simulink model "automata_learning"  (R2022a)
(part 10 of 10)

0.6710054278373718) + 1.0) + 0.26810726523399353 * (exp(0.6629329919815063 * x1 - 0.3119186460971832 * x2 + 0.20862619578838348) - 1.0) / (exp(0.6629329919815063 * x1 - 0.3119186460971832 * x2 + 0.20862619578838348) + 1.0) + 0.9232311844825745 * (exp(0.6406594514846802 * x1 + 0.05703261122107506 * x2 + 0.3176595866680145) - 1.0) / (exp(0.6406594514846802 * x1 + 0.05703261122107506 * x2 + 0.3176595866680145) + 1.0) + 0.7681644558906555 * (exp(0.9188533425331116 * x1 + 0.3101022243499756 * x2 + 0.6654399037361145) - 1.0) / (exp(0.9188533425331116 * x1 + 0.3101022243499756 * x2 + 0.6654399037361145) + 1.0) - 0.2590520679950714 * (exp(0.575993537902832 * x1 - 0.4726734459400177 * x2 + 0.7029635310173035) - 1.0) / (exp(0.575993537902832 * x1 - 0.4726734459400177 * x2 + 0.7029635310173035) + 1.0) + 0.9095823168754578 * (exp(0.7590878009796143 * x1 - 0.23670220375061035 * x2 + 1.0534344911575317) - 1.0) / (exp(0.7590878009796143 * x1 - 0.23670220375061035 * x2 + 1.0534344911575317) + 1.0) + 0.7333047389984131 * (exp(0.5151293277740479 * x1 - 0.39795804023742676 * x2 + 0.11806197464466095) - 1.0) / (exp(0.5151293277740479 * x1 - 0.39795804023742676 * x2 + 0.11806197464466095) + 1.0) + 0.9102956652641296 * (exp(0.4433993697166443 * x1 - 0.08205956220626831 * x2 + 0.18252399563789368) - 1.0) / (exp(0.4433993697166443 * x1 - 0.08205956220626831 * x2 + 0.18252399563789368) + 1.0) + 0.8548353910446167 * (exp(0.48641395568847656 * x1 + 0.8826764822006226 * x2 + 0.5417870879173279) - 1.0) / (exp(0.48641395568847656 * x1 + 0.8826764822006226 * x2 + 0.5417870879173279) + 1.0) + 0.536832332611084 * (exp(0.47229835391044617 * x1 - 0.20287995040416718 * x2 + 0.34894588589668274) - 1.0) / (exp(0.47229835391044617 * x1 - 0.20287995040416718 * x2 + 0.34894588589668274) + 1.0) + 0.24342596530914307) + 1.0) + 0.9671072959899902 * (exp(0.5794932246208191 * (exp(0.55704265832901 * x1 + 0.592957079410553 * x2 + 0.33553701639175415) - 1.0) / (exp(0.55704265832901 * x1 + 0.592957079410553 * x2 + 0.33553701639175415) + 1.0) + 0.9518229365348816 * (exp(0.6549424529075623 * x1 - 0.1391940712928772 * x2 + 0.6311511397361755) - 1.0) / (exp(0.6549424529075623 * x1 - 0.1391940712928772 * x2 + 0.6311511397361755) + 1.0) + 0.44287005066871643 * (exp(0.6888914704322815 * x1 - 0.6110755205154419 * x2 + 0.6041516661643982) - 1.0) / (exp(0.6888914704322815 * x1 - 0.6110755205154419 * x2 + 0.6041516661643982) + 1.0) + 0.6187660694122314 * (exp(0.20129768550395966 * x2 - 1.0647046566009521 * x1 + 0.5778789520263672) - 1.0) / (exp(0.20129768550395966 * x2 - 1.0647046566009521 * x1 + 0.5778789520263672) + 1.0) - 0.48944976925849915 * (exp(0.07980049401521683 * x1 + 0.6124646663665771 * x2 - 0.1684141308069229) - 1.0) / (exp(0.07980049401521683 * x1 + 0.6124646663665771 * x2 - 0.1684141308069229) + 1.0) + 0.1713249534368515 * (exp(0.361889123916626 * x1 + 0.6644142866134644 * x2 + 0.2823045253753662) - 1.0) / (exp(0.361889123916626 * x1 + 0.6644142866134644 * x2 + 0.2823045253753662) + 1.0) - 0.9707628488540649 * (exp(0.6355613470077515 * x1 + 0.7923728823661804 * x2 + 0.27106547355651855) - 1.0) / (exp(0.6355613470077515 * x1 + 0.7923728823661804 * x2 + 0.27106547355651855) + 1.0) + 0.23367302119731903 * (exp(0.2957508862018585 * x1 + 0.41109827160835266 * x2 + 0.13971224427223206) - 1.0) / (exp(0.2957508862018585 * x1 + 0.41109827160835266 * x2 + 0.13971224427223206) + 1.0) - 1.041667103767395 * (exp(0.7331780195236206 * x1 + 1.0149563550949097 * x2 - 0.37788793444633484) - 1.0) / (exp(0.7331780195236206 * x1 + 1.0149563550949097 * x2 - 0.37788793444633484) + 1.0) + 0.5859559774398804 * (exp(0.6101927757263184 * x1 - 0.32282912731170654 * x2 + 0.7518836855888367) - 1.0) / (exp(0.6101927757263184 * x1 - 0.32282912731170654 * x2 + 0.7518836855888367) + 1.0) + 0.6447692513465881 * (exp(0.2542825937271118 * x1 + 0.9084843397140503 * x2 + 0.6710054278373718) - 1.0) / (exp(0.2542825937271118 * x1 + 0.9084843397140503 * x2 + 0.6710054278373718) + 1.0) + 0.8346514701843262 * (exp(0.6629329919815063 * x1 - 0.3119186460971832 * x2 + 0.20862619578838348) - 1.0) / (exp(0.6629329919815063 * x1 - 0.3119186460971832 * x2 + 0.20862619578838348) + 1.0) - 0.11273422837257385 * (exp(0.6406594514846802 * x1 + 0.05703261122107506 * x2 + 0.3176595866680145) - 1.0) / (exp(0.6406594514846802 * x1 + 0.05703261122107506 * x2 + 0.3176595866680145) + 1.0) + 1.3257321119308472 * (exp(0.9188533425331116 * x1 + 0.3101022243499756 * x2 + 0.6654399037361145) - 1.0) / (exp(0.9188533425331116 * x1 + 0.3101022243499756 * x2 + 0.6654399037361145) + 1.0) + 0.364542692899704 * (exp(0.575993537902832 * x1 - 0.4726734459400177 * x2 + 0.7029635310173035) - 1.0) / (exp(0.575993537902832 * x1 - 0.4726734459400177 * x2 + 0.7029635310173035) + 1.0) + 1.3769431114196777 * (exp(0.7590878009796143 * x1 - 0.23670220375061035 * x2 + 1.0534344911575317) - 1.0) / (exp(0.7590878009796143 * x1 - 0.23670220375061035 * x2 + 1.0534344911575317) + 1.0) + 0.25804296135902405 * (exp(0.5151293277740479 * x1 - 0.39795804023742676 * x2 + 0.11806197464466095) - 1.0) / (exp(0.5151293277740479 * x1 - 0.39795804023742676 * x2 + 0.11806197464466095) + 1.0) + 0.17459556460380554 * (exp(0.4433993697166443 * x1 - 0.08205956220626831 * x2 + 0.18252399563789368) - 1.0) / (exp(0.4433993697166443 * x1 - 0.08205956220626831 * x2 + 0.18252399563789368) + 1.0) + 0.7206000089645386 * (exp(0.48641395568847656 * x1 + 0.8826764822006226 * x2 + 0.5417870879173279) - 1.0) / (exp(0.48641395568847656 * x1 + 0.8826764822006226 * x2 + 0.5417870879173279) + 1.0) + 0.03906390815973282 * (exp(0.47229835391044617 * x1 - 0.20287995040416718 * x2 + 0.34894588589668274) - 1.0) / (exp(0.47229835391044617 * x1 - 0.20287995040416718 * x2 + 0.34894588589668274) + 1.0) + 0.22301727533340454) - 1.0) / (exp(0.5794932246208191 * (exp(0.55704265832901 * x1 + 0.592957079410553 * x2 + 0.33553701639175415) - 1.0) / (exp(0.55704265832901 * x1 + 0.592957079410553 * x2 + 0.33553701639175415) + 1.0) + 0.9518229365348816 * (exp(0.6549424529075623 * x1 - 0.1391940712928772 * x2 + 0.6311511397361755) - 1.0) / (exp(0.6549424529075623 * x1 - 0.1391940712928772 * x2 + 0.6311511397361755) + 1.0) + 0.44287005066871643 * (exp(0.6888914704322815 * x1 - 0.6110755205154419 * x2 + 0.6041516661643982) - 1.0) / (exp(0.6888914704322815 * x1 - 0.6110755205154419 * x2 + 0.6041516661643982) + 1.0) + 0.6187660694122314 * (exp(0.20129768550395966 * x2 - 1.0647046566009521 * x1 + 0.5778789520263672) - 1.0) / (exp(0.20129768550395966 * x2 - 1.0647046566009521 * x1 + 0.5778789520263672) + 1.0) - 0.48944976925849915 * (exp(0.07980049401521683 * x1 + 0.6124646663665771 * x2 - 0.1684141308069229) - 1.0) / (exp(0.07980049401521683 * x1 + 0.6124646663665771 * x2 - 0.1684141308069229) + 1.0) + 0.1713249534368515 * (exp(0.361889123916626 * x1 + 0.6644142866134644 * x2 + 0.2823045253753662) - 1.0) / (exp(0.361889123916626 * x1 + 0.6644142866134644 * x2 + 0.2823045253753662) + 1.0) - 0.9707628488540649 * (exp(0.6355613470077515 * x1 + 0.7923728823661804 * x2 + 0.27106547355651855) - 1.0) / (exp(0.6355613470077515 * x1 + 0.7923728823661804 * x2 + 0.27106547355651855) + 1.0) + 0.23367302119731903 * (exp(0.2957508862018585 * x1 + 0.41109827160835266 * x2 + 0.13971224427223206) - 1.0) / (exp(0.2957508862018585 * x1 + 0.41109827160835266 * x2 + 0.13971224427223206) + 1.0) - 1.041667103767395 * (exp(0.7331780195236206 * x1 + 1.0149563550949097 * x2 - 0.37788793444633484) - 1.0) / (exp(0.7331780195236206 * x1 + 1.0149563550949097 * x2 - 0.37788793444633484) + 1.0) + 0.5859559774398804 * (exp(0.6101927757263184 * x1 - 0.32282912731170654 * x2 + 0.7518836855888367) - 1.0) / (exp(0.6101927757263184 * x1 - 0.32282912731170654 * x2 + 0.7518836855888367) + 1.0) + 0.6447692513465881 * (exp(0.2542825937271118 * x1 + 0.9084843397140503 * x2 + 0.6710054278373718) - 1.0) / (exp(0.2542825937271118 * x1 + 0.9084843397140503 * x2 + 0.6710054278373718) + 1.0) + 0.8346514701843262 * (exp(0.6629329919815063 * x1 - 0.3119186460971832 * x2 + 0.20862619578838348) - 1.0) / (exp(0.6629329919815063 * x1 - 0.3119186460971832 * x2 + 0.20862619578838348) + 1.0) - 0.11273422837257385 * (exp(0.6406594514846802 * x1 + 0.05703261122107506 * x2 + 0.3176595866680145) - 1.0) / (exp(0.6406594514846802 * x1 + 0.05703261122107506 * x2 + 0.3176595866680145) + 1.0) + 1.3257321119308472 * (exp(0.9188533425331116 * x1 + 0.3101022243499756 * x2 + 0.6654399037361145) - 1.0) / (exp(0.9188533425331116 * x1 + 0.3101022243499756 * x2 + 0.6654399037361145) + 1.0) + 0.364542692899704 * (exp(0.575993537902832 * x1 - 0.4726734459400177 * x2 + 0.7029635310173035) - 1.0) / (exp(0.575993537902832 * x1 - 0.4726734459400177 * x2 + 0.7029635310173035) + 1.0) + 1.3769431114196777 * (exp(0.7590878009796143 * x1 - 0.23670220375061035 * x2 + 1.0534344911575317) - 1.0) / (exp(0.7590878009796143 * x1 - 0.23670220375061035 * x2 + 1.0534344911575317) + 1.0) + 0.25804296135902405 * (exp(0.5151293277740479 * x1 - 0.39795804023742676 * x2 + 0.11806197464466095) - 1.0) / (exp(0.5151293277740479 * x1 - 0.39795804023742676 * x2 + 0.11806197464466095) + 1.0) + 0.17459556460380554 * (exp(0.4433993697166443 * x1 - 0.08205956220626831 * x2 + 0.18252399563789368) - 1.0) / (exp(0.4433993697166443 * x1 - 0.08205956220626831 * x2 + 0.18252399563789368) + 1.0) + 0.7206000089645386 * (exp(0.48641395568847656 * x1 + 0.8826764822006226 * x2 + 0.5417870879173279) - 1.0) / (exp(0.48641395568847656 * x1 + 0.8826764822006226 * x2 + 0.5417870879173279) + 1.0) + 0.03906390815973282 * (exp(0.47229835391044617 * x1 - 0.20287995040416718 * x2 + 0.34894588589668274) - 1.0) / (exp(0.47229835391044617 * x1 - 0.20287995040416718 * x2 + 0.34894588589668274) + 1.0) + 0.22301727533340454) + 1.0) + 0.44379422068595886 * (exp(0.004474600311368704 * (exp(0.6549424529075623 * x1 - 0.1391940712928772 * x2 + 0.6311511397361755) - 1.0) / (exp(0.6549424529075623 * x1 - 0.1391940712928772 * x2 + 0.6311511397361755) + 1.0) - 0.22987298667430878 * (exp(0.55704265832901 * x1 + 0.592957079410553 * x2 + 0.33553701639175415) - 1.0) / (exp(0.55704265832901 * x1 + 0.592957079410553 * x2 + 0.33553701639175415) + 1.0) + 0.6058520674705505 * (exp(0.6888914704322815 * x1 - 0.6110755205154419 * x2 + 0.6041516661643982) - 1.0) / (exp(0.6888914704322815 * x1 - 0.6110755205154419 * x2 + 0.6041516661643982) + 1.0) - 1.357459306716919 * (exp(0.20129768550395966 * x2 - 1.0647046566009521 * x1 + 0.5778789520263672) - 1.0) / (exp(0.20129768550395966 * x2 - 1.0647046566009521 * x1 + 0.5778789520263672) + 1.0) - 0.15493887662887573 * (exp(0.07980049401521683 * x1 + 0.6124646663665771 * x2 - 0.1684141308069229) - 1.0) / (exp(0.07980049401521683 * x1 + 0.6124646663665771 * x2 - 0.1684141308069229) + 1.0) + 0.5729637742042542 * (exp(0.361889123916626 * x1 + 0.6644142866134644 * x2 + 0.2823045253753662) - 1.0) / (exp(0.361889123916626 * x1 + 0.6644142866134644 * x2 + 0.2823045253753662) + 1.0) + 0.14763222634792328 * (exp(0.6355613470077515 * x1 + 0.7923728823661804 * x2 + 0.27106547355651855) - 1.0) / (exp(0.6355613470077515 * x1 + 0.7923728823661804 * x2 + 0.27106547355651855) + 1.0) + 0.9889805912971497 * (exp(0.2957508862018585 * x1 + 0.41109827160835266 * x2 + 0.13971224427223206) - 1.0) / (exp(0.2957508862018585 * x1 + 0.41109827160835266 * x2 + 0.13971224427223206) + 1.0) - 0.027431178838014603 * (exp(0.7331780195236206 * x1 + 1.0149563550949097 * x2 - 0.37788793444633484) - 1.0) / (exp(0.7331780195236206 * x1 + 1.0149563550949097 * x2 - 0.37788793444633484) + 1.0) - 0.22922979295253754 * (exp(0.6101927757263184 * x1 - 0.32282912731170654 * x2 + 0.7518836855888367) - 1.0) / (exp(0.6101927757263184 * x1 - 0.32282912731170654 * x2 + 0.7518836855888367) + 1.0) + 0.16280798614025116 * (exp(0.2542825937271118 * x1 + 0.9084843397140503 * x2 + 0.6710054278373718) - 1.0) / (exp(0.2542825937271118 * x1 + 0.9084843397140503 * x2 + 0.6710054278373718) + 1.0) + 0.3429515063762665 * (exp(0.6629329919815063 * x1 - 0.3119186460971832 * x2 + 0.20862619578838348) - 1.0) / (exp(0.6629329919815063 * x1 - 0.3119186460971832 * x2 + 0.20862619578838348) + 1.0) + 1.2585675716400146 * (exp(0.6406594514846802 * x1 + 0.05703261122107506 * x2 + 0.3176595866680145) - 1.0) / (exp(0.6406594514846802 * x1 + 0.05703261122107506 * x2 + 0.3176595866680145) + 1.0) + 0.7193031311035156 * (exp(0.9188533425331116 * x1 + 0.3101022243499756 * x2 + 0.6654399037361145) - 1.0) / (exp(0.9188533425331116 * x1 + 0.3101022243499756 * x2 + 0.6654399037361145) + 1.0) + 0.42601025104522705 * (exp(0.575993537902832 * x1 - 0.4726734459400177 * x2 + 0.7029635310173035) - 1.0) / (exp(0.575993537902832 * x1 - 0.4726734459400177 * x2 + 0.7029635310173035) + 1.0) + 0.8000105023384094 * (exp(0.7590878009796143 * x1 - 0.23670220375061035 * x2 + 1.0534344911575317) - 1.0) / (exp(0.7590878009796143 * x1 - 0.23670220375061035 * x2 + 1.0534344911575317) + 1.0) + 0.8869855999946594 * (exp(0.5151293277740479 * x1 - 0.39795804023742676 * x2 + 0.11806197464466095) - 1.0) / (exp(0.5151293277740479 * x1 - 0.39795804023742676 * x2 + 0.11806197464466095) + 1.0) + 0.6011543273925781 * (exp(0.4433993697166443 * x1 - 0.08205956220626831 * x2 + 0.18252399563789368) - 1.0) / (exp(0.4433993697166443 * x1 - 0.08205956220626831 * x2 + 0.18252399563789368) + 1.0) - 0.04096032679080963 * (exp(0.48641395568847656 * x1 + 0.8826764822006226 * x2 + 0.5417870879173279) - 1.0) / (exp(0.48641395568847656 * x1 + 0.8826764822006226 * x2 + 0.5417870879173279) + 1.0) + 0.8472379446029663 * (exp(0.47229835391044617 * x1 - 0.20287995040416718 * x2 + 0.34894588589668274) - 1.0) / (exp(0.47229835391044617 * x1 - 0.20287995040416718 * x2 + 0.34894588589668274) + 1.0) - 0.481460839509964) - 1.0) / (exp(0.004474600311368704 * (exp(0.6549424529075623 * x1 - 0.1391940712928772 * x2 + 0.6311511397361755) - 1.0) / (exp(0.6549424529075623 * x1 - 0.1391940712928772 * x2 + 0.6311511397361755) + 1.0) - 0.22987298667430878 * (exp(0.55704265832901 * x1 + 0.592957079410553 * x2 + 0.33553701639175415) - 1.0) / (exp(0.55704265832901 * x1 + 0.592957079410553 * x2 + 0.33553701639175415) + 1.0) + 0.6058520674705505 * (exp(0.6888914704322815 * x1 - 0.6110755205154419 * x2 + 0.6041516661643982) - 1.0) / (exp(0.6888914704322815 * x1 - 0.6110755205154419 * x2 + 0.6041516661643982) + 1.0) - 1.357459306716919 * (exp(0.20129768550395966 * x2 - 1.0647046566009521 * x1 + 0.5778789520263672) - 1.0) / (exp(0.20129768550395966 * x2 - 1.0647046566009521 * x1 + 0.5778789520263672) + 1.0) - 0.15493887662887573 * (exp(0.07980049401521683 * x1 + 0.6124646663665771 * x2 - 0.1684141308069229) - 1.0) / (exp(0.07980049401521683 * x1 + 0.6124646663665771 * x2 - 0.1684141308069229) + 1.0) + 0.5729637742042542 * (exp(0.361889123916626 * x1 + 0.6644142866134644 * x2 + 0.2823045253753662) - 1.0) / (exp(0.361889123916626 * x1 + 0.6644142866134644 * x2 + 0.2823045253753662) + 1.0) + 0.14763222634792328 * (exp(0.6355613470077515 * x1 + 0.7923728823661804 * x2 + 0.27106547355651855) - 1.0) / (exp(0.6355613470077515 * x1 + 0.7923728823661804 * x2 + 0.27106547355651855) + 1.0) + 0.9889805912971497 * (exp(0.2957508862018585 * x1 + 0.41109827160835266 * x2 + 0.13971224427223206) - 1.0) / (exp(0.2957508862018585 * x1 + 0.41109827160835266 * x2 + 0.13971224427223206) + 1.0) - 0.027431178838014603 * (exp(0.7331780195236206 * x1 + 1.0149563550949097 * x2 - 0.37788793444633484) - 1.0) / (exp(0.7331780195236206 * x1 + 1.0149563550949097 * x2 - 0.37788793444633484) + 1.0) - 0.22922979295253754 * (exp(0.6101927757263184 * x1 - 0.32282912731170654 * x2 + 0.7518836855888367) - 1.0) / (exp(0.6101927757263184 * x1 - 0.32282912731170654 * x2 + 0.7518836855888367) + 1.0) + 0.16280798614025116 * (exp(0.2542825937271118 * x1 + 0.9084843397140503 * x2 + 0.6710054278373718) - 1.0) / (exp(0.2542825937271118 * x1 + 0.9084843397140503 * x2 + 0.6710054278373718) + 1.0) + 0.3429515063762665 * (exp(0.6629329919815063 * x1 - 0.3119186460971832 * x2 + 0.20862619578838348) - 1.0) / (exp(0.6629329919815063 * x1 - 0.3119186460971832 * x2 + 0.20862619578838348) + 1.0) + 1.2585675716400146 * (exp(0.6406594514846802 * x1 + 0.05703261122107506 * x2 + 0.3176595866680145) - 1.0) / (exp(0.6406594514846802 * x1 + 0.05703261122107506 * x2 + 0.3176595866680145) + 1.0) + 0.7193031311035156 * (exp(0.9188533425331116 * x1 + 0.3101022243499756 * x2 + 0.6654399037361145) - 1.0) / (exp(0.9188533425331116 * x1 + 0.3101022243499756 * x2 + 0.6654399037361145) + 1.0) + 0.42601025104522705 * (exp(0.575993537902832 * x1 - 0.4726734459400177 * x2 + 0.7029635310173035) - 1.0) / (exp(0.575993537902832 * x1 - 0.4726734459400177 * x2 + 0.7029635310173035) + 1.0) + 0.8000105023384094 * (exp(0.7590878009796143 * x1 - 0.23670220375061035 * x2 + 1.0534344911575317) - 1.0) / (exp(0.7590878009796143 * x1 - 0.23670220375061035 * x2 + 1.0534344911575317) + 1.0) + 0.8869855999946594 * (exp(0.5151293277740479 * x1 - 0.39795804023742676 * x2 + 0.11806197464466095) - 1.0) / (exp(0.5151293277740479 * x1 - 0.39795804023742676 * x2 + 0.11806197464466095) + 1.0) + 0.6011543273925781 * (exp(0.4433993697166443 * x1 - 0.08205956220626831 * x2 + 0.18252399563789368) - 1.0) / (exp(0.4433993697166443 * x1 - 0.08205956220626831 * x2 + 0.18252399563789368) + 1.0) - 0.04096032679080963 * (exp(0.48641395568847656 * x1 + 0.8826764822006226 * x2 + 0.5417870879173279) - 1.0) / (exp(0.48641395568847656 * x1 + 0.8826764822006226 * x2 + 0.5417870879173279) + 1.0) + 0.8472379446029663 * (exp(0.47229835391044617 * x1 - 0.20287995040416718 * x2 + 0.34894588589668274) - 1.0) / (exp(0.47229835391044617 * x1 - 0.20287995040416718 * x2 + 0.34894588589668274) + 1.0) - 0.481460839509964) + 1.0) - 0.11512385308742523;
    x1_out=x1;
    x2_out=x2;
    automata_learning_location =2;
  loc1 -> loc2 : [0.3288 * x1 - 0.333 * x2 + 1.0 < 0.0]
  (default) -> loc1 : {x1 = 1.0;
      | x2 = -1.0;}
  loc2 -> loc1 : [0.499 * x2 - 0.0006802 * x1 + 1.0 < 0.0]
  data: x1_out output; x1 local; x2_out output; x2 local; automata_learning_location output
  data x1 settings: updateMethod=SF_CONTINUOUS_TIME_DATA
  data x2 settings: updateMethod=SF_CONTINUOUS_TIME_DATA
